simulink model "D3"  (R2017a)
settings: Solver=VariableStepAuto  StartTime=0.0  StopTime=1  RelTol=1e-3
settings Model: Creator=wuyuche3  LastModifiedBy=wuyuche3

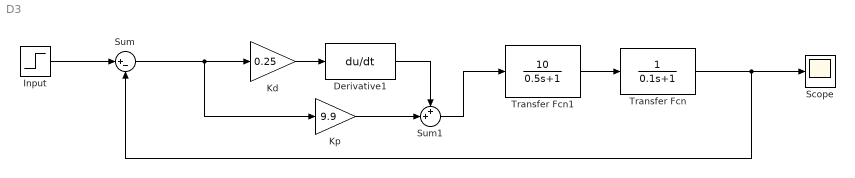
== system D3 ==
  Derivative1 : Derivative  CoefficientInTFapproximation=0
  Input : Step  Time=0  SampleTime=0
  "Kd " : Gain  Gain=0.25
  Kp : Gain  Gain=9.9
  Scope : Scope
  Sum : Sum  Inputs=|+-
  Sum1 : Sum  Inputs=++|
  Transfer Fcn : TransferFcn  Denominator=[0.1 1]
  Transfer Fcn1 : TransferFcn  Numerator=[10]  Denominator=[0.5 1]
  wires:
  Transfer Fcn/1 -> Scope/1, Sum/2
  Sum1/1 -> Transfer Fcn1/1
  Kp/1 -> Sum1/2
  Transfer Fcn1/1 -> Transfer Fcn/1
  "Kd "/1 -> Derivative1/1
  Derivative1/1 -> Sum1/1
  Input/1 -> Sum/1
  Sum/1 -> Kp/1, "Kd "/1
